simulink model "GFL_Control"  (R2025a)
settings: Solver=FixedStepDiscrete  StartTime=0.0  StopTime=10.0  RelTol=1e-3
undefined symbols (not defined in the file or in its folder): CheckSeconds, Curr_Controllor_Ki, Curr_Controllor_Kp, Curr_Controllor_Max, Curr_Controllor_Min, CurrPIDLimits4d, CurrPIDParams4d, DiscIntNeverNeededParam, MaxGridVolt, MaxGridwFreq, MaxUdcVolt, MinGridwFreq, MinUdcVolt, PLL_f0, PLL_Init_Theta, PLL_Ki, PLL_Kp
libraries: slpidlib x3, spsabctodq0Lib x2, spsdq0toabcLib x1
settings Model: Creator=yucha  LastModifiedBy=yucha
settings OptimizationCC: DefaultParameterBehavior=Inlined  EnhancedBackFolding=on  PassReuseOutputArgsAs=Individual arguments  ZeroExternalMemoryAtStartup=off  ZeroInternalMemoryAtStartup=off  OptimizeBlockOrder=speed  DifferentSizesBufferReuse=on  OptimizationCustomize=off  EfficientTunableParamExpr=on
settings DebuggingCC: ParameterTunabilityLossMsg=error
settings HardwareCC: TargetBitPerPointer=64.0  TargetBitPerSizeT=64.0  TargetBitPerPtrDiffT=64.0  TargetLongLongMode=on  TargetIntDivRoundTo=Zero  TargetEndianess=LittleEndian  TargetWordSize=64.0  TargetHWDeviceType=MATLAB Host  ProdEqTarget=off
settings SFSimCC: MATLABDynamicMemAlloc=off
settings RTWCC: SystemTargetFile=ert_shrlib.tlc  TemplateMakefile=ert_default_tmf  Description=Embedded Coder (host-based shared library target)
settings CodeAppCC: ForceParamTrailComments=on  IgnoreCustomStorageClasses=off  OperatorAnnotations=on  SimulinkDataObjDesc=on  SFDataObjDesc=on  InsertBlockDesc=on
settings STFCustomTargetCC: SystemTargetFile=ert_shrlib.tlc  TargetLangStandard=C99 (ISO)  MultiwordLength=256.0  DynamicStringBufferSize=256.0  GenerateSampleERTMain=on  ParMdlRefBuildCompliant=on  CompOptLevelCompliant=on  CombineOutputUpdateFcns=on  ERTCustomFileBanners=on  SupportContinuousTime=off  SupportNonInlinedSFcns=off  RemoveResetFunc=on  MATLABClassNameForMDSCustomization=Simulink.SoftwareTarget.ERTCustomization  ModelStepFunctionPrototypeControlCompliant=on  GRTInterface=off  UseToolchainInfoCompliant=on
settings ERTTargetCC: ExtModeTransport=0.0  ExtModeStaticAlloc=off  ExtModeMexFile=ext_comm  ExtModeIntrfLevel=Level1  ERTCustomFileTemplate=example_file_process.tlc  TargetLangStandard=C99 (ISO)  GenerateSampleERTMain=on  ConcurrentExecutionCompliant=off  CPPClassGenCompliant=off

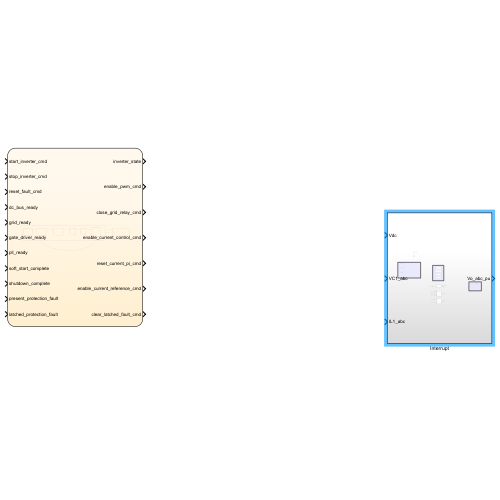
[thumbnail: Simulink's stored preview of the top-level diagram]
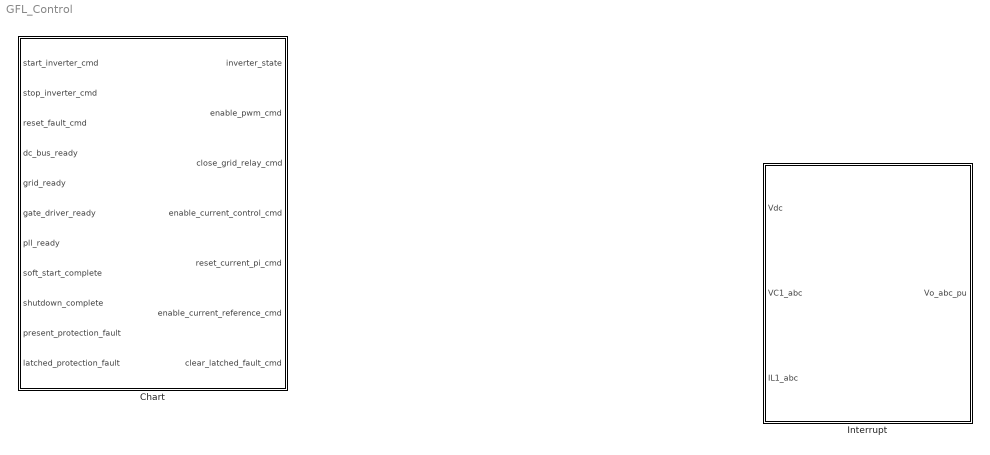
== system GFL_Control ==
  Chart : Stateflow chart  TreatAsAtomicUnit=on
  Interrupt : Subsystem

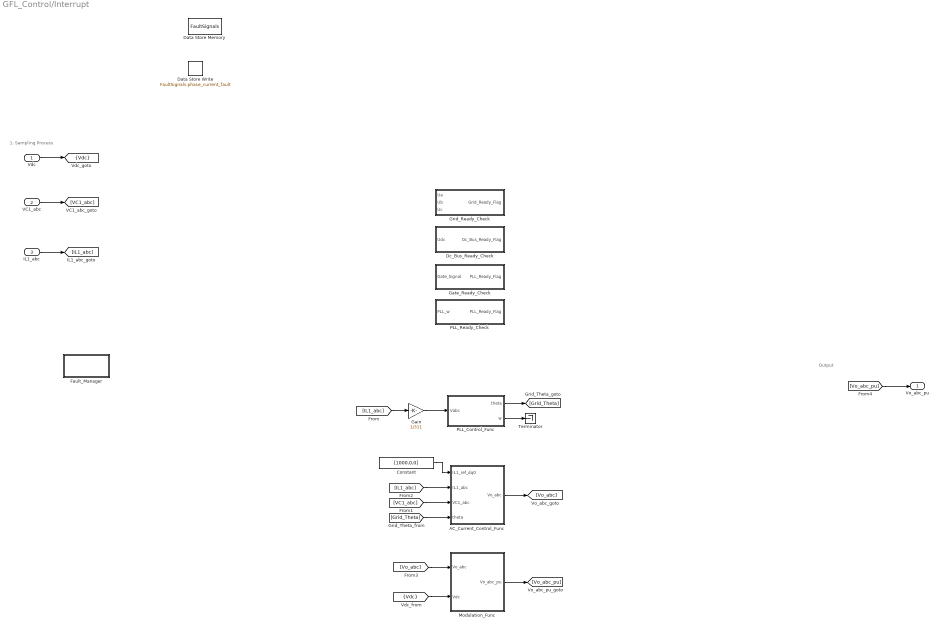
== system GFL_Control/Interrupt ==
  note: 1. Sampling Process
  note: Output
  Vdc : Inport
  VC1_abc : Inport  Port=2
  IL1_abc : Inport  Port=3
  AC_Current_Control_Func : Subsystem  InitFcn=|
      | Curr_Controller_Kp = 1;
      | Curr_Controller_Ki = 1000;
      | Curr_Controller_max = 200;
      | Curr_Controller_min = -200;
  Constant : Constant  Value=[1000,0,0]
  Data Store Memory : DataStoreMemory  DataStoreName=FaultSignals  WriteAfterWriteMsg=warning  ShowAdditionalParam=off  OutDataTypeStr=Bus: FaultSignalsStruct
  Data Store Write : DataStoreWrite  DataStoreName=FaultSignals  DataStoreElements=FaultSignals.phase_current_fault  IndexOptions=Index vector (dialog)  Indices=1  OutputSizes=1
  Dc_Bus_Ready_Check : Subsystem  InitFcn=|
      | MaxUdcVolt = 1200;
      | MinUdcVolt = 650;
      | CheckSeconds = 1;
  Fault_Manager : Subsystem
  Gain : Gain  Gain=1/311
  Gate_Ready_Check : Subsystem  InitFcn=CheckSeconds = 1;
  Grid_Ready_Check : Subsystem
  Modulation_Func : Subsystem  InitFcn=|
      | Curr_Controller_Kp = 1;
      | Curr_Controller_Ki = 1000;
      | Curr_Controller_max = 200;
      | Curr_Controller_min = -200;
  PLL_Control_Func : Subsystem  InitFcn=|
      | PLL_Controller_Kp = 166.0;
      | PLL_Controller_Ki = 25550.0;
      | PLL_Init_Theta = 0;
      | PLL_f0 = 50.0;
  PLL_Ready_Check : Subsystem  InitFcn=|
      | MaxGridwFreq = 100*pi*1.1;
      | MinGridwFreq = 100*pi*0.9;
      | CheckSeconds = 1;
  Terminator : Terminator
  Vo_abc_pu : Outport
  tag scope: Vdc=scoped
  wires:
  VC1_abc/1 -> [VC1_abc]
  IL1_abc/1 -> [IL1_abc]
  Vdc/1 -> [Vdc]
  PLL_Control_Func/2(w) -> Terminator/1
  [Vdc] -> Modulation_Func/2(Vdc)
  Gain/1 -> PLL_Control_Func/1(Vabc)
  [IL1_abc] -> AC_Current_Control_Func/2(IL1_abc)
  [Grid_Theta] -> AC_Current_Control_Func/4(theta)
  [IL1_abc] -> Gain/1
  PLL_Control_Func/1(theta) -> [Grid_Theta]
  [Vo_abc] -> Modulation_Func/1(Vo_abc)
  AC_Current_Control_Func/1(Vo_abc) -> [Vo_abc]
  Modulation_Func/1(Vo_abc_pu) -> [Vo_abc_pu]
  [VC1_abc] -> AC_Current_Control_Func/3(VC1_abc)
  Constant/1 -> AC_Current_Control_Func/1(IL1_ref_dq0)
  [Vo_abc_pu] -> Vo_abc_pu/1

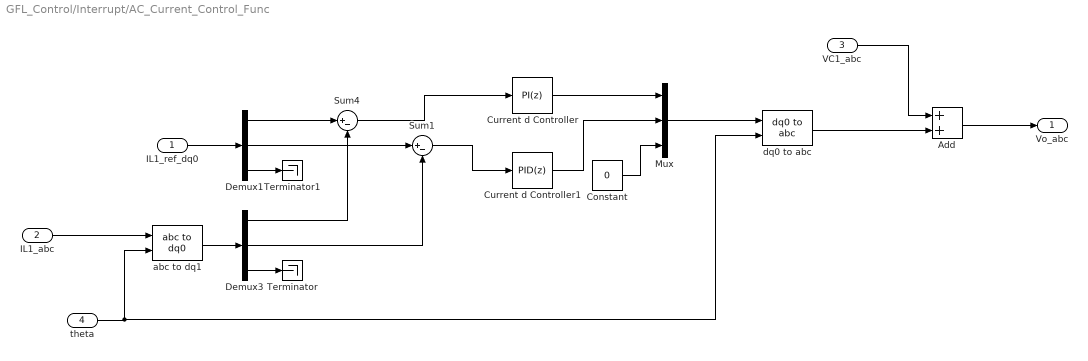
== system GFL_Control/Interrupt/AC_Current_Control_Func ==
  IL1_ref_dq0 : Inport
  IL1_abc : Inport  Port=2
  VC1_abc : Inport  Port=3
  theta : Inport  Port=4
  Add : Sum
  Constant : Constant  Value=0
  Current d Controller : slpidlib/PID Controller  Controller=PI  Form=Parallel  TimeDomain=Discrete-time  UseExternalTs=off  SampleTime=-1  IntegratorMethod=Forward Euler  FilterMethod=Forward Euler  ControllerParametersSource=internal  P=Curr_Controllor_Kp  I=Curr_Controllor_Ki  UseKiTs=on  D=CurrPIDParams4d(3)  UseExternalDerivativeSource=off  N=100  UseFilter=on  TunerSelectOption=Transfer Function Based (PID Tuner App)  InitialConditionSource=internal  InitialConditionForIntegrator=0  InitialConditionForFilter=0  DifferentiatorICPrevScaledInput=0  ExternalReset=none  TrackingMode=off  Kt=1  LimitOutput=on  SatLimitsSource=internal  UpperSaturationLimit=Curr_Controllor_Max  LowerSaturationLimit=Curr_Controllor_Min  LinearizeAsGain=off  AntiWindupMode=clamping  Kb=1  LimitIntegrator=off  UpperIntegratorSaturationLimit=inf  LowerIntegratorSaturationLimit=-inf  POutMin=[]  POutMax=[]  IOutMin=[]  IOutMax=[]  DOutMin=[]  DOutMax=[]  NOutMin=[]  NOutMax=[]  SumOutMin=[]  SumOutMax=[]  SaturationOutMin=[]  SaturationOutMax=[]  PParamMin=[]  PParamMax=[]  IParamMin=[]  IParamMax=[]  DParamMin=[]  DParamMax=[]  NParamMin=[]  NParamMax=[]  KbParamMin=[]  KbParamMax=[]  KtParamMin=[]  KtParamMax=[]  KbOutMin=[]  KbOutMax=[]  KtOutMin=[]  KtOutMax=[]  IntegratorOutMin=[]  IntegratorOutMax=[]  FilterOutMin=[]  FilterOutMax=[]  SumI1OutMin=[]  SumI1OutMax=[]  SumI2OutMin=[]  SumI2OutMax=[]  SumI3OutMin=[]  SumI3OutMax=[]  SumI4OutMin=[]  SumI4OutMax=[]  SumDOutMin=[]  SumDOutMax=[]  DifferentiatorOutMin=[]  DifferentiatorOutMax=[]  FilterDiffOutCoefMin=[]  FilterDiffOutCoefMax=[]  ReciprocalOutMin=[]  ReciprocalOutMax=[]  SumDenOutMin=[]  SumDenOutMax=[]  SumNumOutMin=[]  SumNumOutMax=[]  DivideOutMin=[]  DivideOutMax=[]  UdiffTsProdOutMin=[]  UdiffTsProdOutMax=[]  NTsProdOutMin=[]  NTsProdOutMax=[]  UintegralTsProdOutMin=[]  UintegralTsProdOutMax=[]  UngainTsProdOutMin=[]  UngainTsProdOutMax=[]  ClampingZeroOutDataTypeStr=Inherit: Inherit via back propagation  ClampingZeroOutMin=[]  ClampingZeroOutMax=[]  FilterDenConstantOutDataTypeStr=Inherit: Inherit via back propagation  FilterDenConstantOutMin=[]  FilterDenConstantOutMax=[]  PCopyOutDataTypeStr=Inherit: Inherit via back propagation  PCopyOutMin=[]  PCopyOutMax=[]  NCopyOutDataTypeStr=Inherit: Inherit via back propagation  NCopyOutMin=[]  NCopyOutMax=[]  IntegratorContinuousStateAttributes=''  IntegratorStateMustResolveToSignalObject=off  IntegratorRTWStateStorageClass=Auto  FilterContinuousStateAttributes=''  FilterStateMustResolveToSignalObject=off  FilterRTWStateStorageClass=Auto  ParallelPVariant=InternalParameters  IdealPVariant=Disabled  IVariant=InternalParameters  DVariant=Disabled  IntegratorVariant=Discrete  SatVariant=Enabled  AWVariant=DiscClampingParallel  PCopyVariant=Disabled  TRVariant=Disabled  FdbkBlocksVariant=Forward  IdealPFdbkVariant=Disabled  SatFdbkVariant=Disabled  DerivativeFilterVariant=Disabled  NVariant=Disabled  NCopyVariant=Disabled_SignalSpec  FilterICVariant=Disabled  IntegratorICVariant=InternalICs  ExternalResetVariant=Disabled  TRSumVariant=Passthrough  SumFdbkVariant=Disabled  SumVariant=Sum_PI  TsampFilterVariant=InternalTs  TsampNgainVariant=Passthrough  TsampIntegralVariant=Disabled_SignalSpec  ExternalSaturationOutDataTypeStr=Inherit: Same as second input  DerivativeSourceVariant=Disabled  PreIntVariant=InternalPreInt
      settings: LibrarySourceBlock=simulink/Discrete/Discrete PID Controller
  Current d Controller1 : slpidlib/PID Controller  Controller=PID  Form=Parallel  TimeDomain=Discrete-time  UseExternalTs=off  SampleTime=-1  IntegratorMethod=Forward Euler  FilterMethod=Forward Euler  ControllerParametersSource=internal  P=CurrPIDParams4d(1)  I=CurrPIDParams4d(2)  UseKiTs=off  D=CurrPIDParams4d(3)  UseExternalDerivativeSource=off  N=100  UseFilter=on  TunerSelectOption=Transfer Function Based (PID Tuner App)  InitialConditionSource=internal  InitialConditionForIntegrator=0  InitialConditionForFilter=0  DifferentiatorICPrevScaledInput=0  ExternalReset=none  TrackingMode=off  Kt=1  LimitOutput=on  SatLimitsSource=internal  UpperSaturationLimit=CurrPIDLimits4d(2)  LowerSaturationLimit=CurrPIDLimits4d(1)  LinearizeAsGain=off  AntiWindupMode=clamping  Kb=1  LimitIntegrator=off  UpperIntegratorSaturationLimit=inf  LowerIntegratorSaturationLimit=-inf  POutMin=[]  POutMax=[]  IOutMin=[]  IOutMax=[]  DOutMin=[]  DOutMax=[]  NOutMin=[]  NOutMax=[]  SumOutMin=[]  SumOutMax=[]  SaturationOutMin=[]  SaturationOutMax=[]  PParamMin=[]  PParamMax=[]  IParamMin=[]  IParamMax=[]  DParamMin=[]  DParamMax=[]  NParamMin=[]  NParamMax=[]  KbParamMin=[]  KbParamMax=[]  KtParamMin=[]  KtParamMax=[]  KbOutMin=[]  KbOutMax=[]  KtOutMin=[]  KtOutMax=[]  IntegratorOutMin=[]  IntegratorOutMax=[]  FilterOutMin=[]  FilterOutMax=[]  SumI1OutMin=[]  SumI1OutMax=[]  SumI2OutMin=[]  SumI2OutMax=[]  SumI3OutMin=[]  SumI3OutMax=[]  SumI4OutMin=[]  SumI4OutMax=[]  SumDOutMin=[]  SumDOutMax=[]  DifferentiatorOutMin=[]  DifferentiatorOutMax=[]  FilterDiffOutCoefMin=[]  FilterDiffOutCoefMax=[]  ReciprocalOutMin=[]  ReciprocalOutMax=[]  SumDenOutMin=[]  SumDenOutMax=[]  SumNumOutMin=[]  SumNumOutMax=[]  DivideOutMin=[]  DivideOutMax=[]  UdiffTsProdOutMin=[]  UdiffTsProdOutMax=[]  NTsProdOutMin=[]  NTsProdOutMax=[]  UintegralTsProdOutMin=[]  UintegralTsProdOutMax=[]  UngainTsProdOutMin=[]  UngainTsProdOutMax=[]  ClampingZeroOutDataTypeStr=Inherit: Inherit via back propagation  ClampingZeroOutMin=[]  ClampingZeroOutMax=[]  FilterDenConstantOutDataTypeStr=Inherit: Inherit via back propagation  FilterDenConstantOutMin=[]  FilterDenConstantOutMax=[]  PCopyOutDataTypeStr=Inherit: Inherit via back propagation  PCopyOutMin=[]  PCopyOutMax=[]  NCopyOutDataTypeStr=Inherit: Inherit via back propagation  NCopyOutMin=[]  NCopyOutMax=[]  IntegratorContinuousStateAttributes=''  IntegratorStateMustResolveToSignalObject=off  IntegratorRTWStateStorageClass=Auto  FilterContinuousStateAttributes=''  FilterStateMustResolveToSignalObject=off  FilterRTWStateStorageClass=Auto  ParallelPVariant=InternalParameters  IdealPVariant=Disabled  IVariant=InternalParameters  DVariant=InternalParameters  IntegratorVariant=Discrete  SatVariant=Enabled  AWVariant=DiscClampingParallel  PCopyVariant=Disabled  TRVariant=Disabled  FdbkBlocksVariant=Forward  IdealPFdbkVariant=Disabled  SatFdbkVariant=Disabled  DerivativeFilterVariant=ForwardEulerFilter  NVariant=InternalParameters  NCopyVariant=Disabled  FilterICVariant=InternalICsFilter  IntegratorICVariant=InternalICs  ExternalResetVariant=Disabled  TRSumVariant=Passthrough  SumFdbkVariant=Disabled  SumVariant=Sum_PID  TsampFilterVariant=InternalTs  TsampNgainVariant=Passthrough  TsampIntegralVariant=Disabled_SignalSpec  ExternalSaturationOutDataTypeStr=Inherit: Same as second input  DerivativeSourceVariant=ErrorSignal  PreIntVariant=InternalPreInt
      settings: LibrarySourceBlock=simulink/Discrete/Discrete PID Controller
  Demux1 : Demux  Outputs=3
  Demux3 : Demux  Outputs=3
  Mux : Mux  Inputs=3
  Sum1 : Sum  Inputs=|+-
  Sum4 : Sum  Inputs=|+-
  Terminator : Terminator
  Terminator1 : Terminator
  abc to dq1 : spsabctodq0Lib/abc to dq0  Alignment=Aligned with phase A axis
  dq0 to abc : spsdq0toabcLib/dq0 to abc  Alignment=Aligned with phase A axis
  Vo_abc : Outport
  wires:
  IL1_abc/1 -> abc to dq1/1
  theta/1 -> dq0 to abc/2, abc to dq1/2
  abc to dq1/1 -> Demux3/1
  IL1_ref_dq0/1 -> Demux1/1
  Demux3/3 -> Terminator/1
  Demux1/3 -> Terminator1/1
  Demux1/1 -> Sum4/1
  Demux1/2 -> Sum1/1
  Demux3/1 -> Sum4/2
  Demux3/2 -> Sum1/2
  Sum4/1 -> Current d Controller/1
  Sum1/1 -> Current d Controller1/1
  Current d Controller/1 -> Mux/1
  Current d Controller1/1 -> Mux/2
  Constant/1 -> Mux/3
  Add/1 -> Vo_abc/1
  VC1_abc/1 -> Add/1
  Mux/1 -> dq0 to abc/1
  dq0 to abc/1 -> Add/2

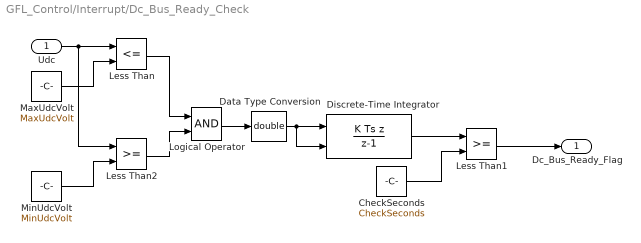
== system GFL_Control/Interrupt/Dc_Bus_Ready_Check ==
  Udc : Inport
  CheckSeconds : Constant  Value=CheckSeconds
  Data Type Conversion : DataTypeConversion  OutDataTypeStr=double  SaturateOnIntegerOverflow=off  RndMeth=Floor
  Discrete-Time Integrator : DiscreteIntegrator  IntegratorMethod=Integration: Backward Euler  ExternalReset=falling  SampleTime=-1  LimitOutput=on  UpperSaturationLimit=100  LowerSaturationLimit=0  ICPrevOutput=DiscIntNeverNeededParam  ICPrevScaledInput=DiscIntNeverNeededParam
  Less Than : RelationalOperator  Operator=<=  OutDataTypeStr=boolean  RndMeth=Simplest  InputSameDT=off
  Less Than1 : RelationalOperator  OutDataTypeStr=boolean  RndMeth=Simplest  InputSameDT=off
  Less Than2 : RelationalOperator  OutDataTypeStr=boolean  RndMeth=Simplest  InputSameDT=off
  Logical Operator : Logic  AllPortsSameDT=off  OutDataTypeStr=boolean
  MaxUdcVolt : Constant  Value=MaxUdcVolt
  MinUdcVolt : Constant  Value=MinUdcVolt
  Dc_Bus_Ready_Flag : Outport
  wires:
  Less Than/1 -> Logical Operator/1
  MaxUdcVolt/1 -> Less Than/2
  CheckSeconds/1 -> Less Than1/2
  Data Type Conversion/1 -> Discrete-Time Integrator/1, Discrete-Time Integrator/2
  Discrete-Time Integrator/1 -> Less Than1/1
  Less Than1/1 -> Dc_Bus_Ready_Flag/1
  Logical Operator/1 -> Data Type Conversion/1
  Udc/1 -> Less Than2/1, Less Than/1
  MinUdcVolt/1 -> Less Than2/2
  Less Than2/1 -> Logical Operator/2

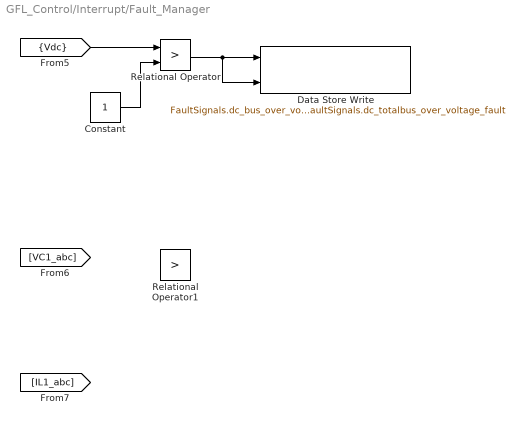
== system GFL_Control/Interrupt/Fault_Manager ==
  Constant : Constant
  Data Store Write : DataStoreWrite  DataStoreName=FaultSignals  DataStoreElements=FaultSignals.dc_bus_over_voltage_fault#FaultSignals.dc_totalbus_over_voltage_fault  IndexOptions=Index vector (dialog)  Indices=1  OutputSizes=1
  Relational Operator : RelationalOperator  Operator=>  OutDataTypeStr=boolean  RndMeth=Simplest  InputSameDT=off
  Relational Operator1 : RelationalOperator  Operator=>  OutDataTypeStr=boolean  RndMeth=Simplest  InputSameDT=off
  wires:
  [Vdc] -> Relational Operator/1
  Constant/1 -> Relational Operator/2
  Relational Operator/1 -> Data Store Write/2, Data Store Write/1

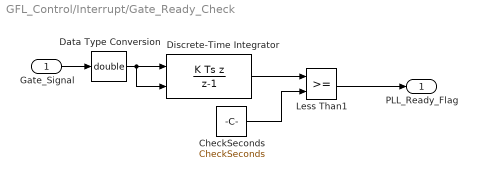
== system GFL_Control/Interrupt/Gate_Ready_Check ==
  Gate_Signal : Inport
  CheckSeconds : Constant  Value=CheckSeconds
  Data Type Conversion : DataTypeConversion  OutDataTypeStr=double  SaturateOnIntegerOverflow=off  RndMeth=Floor
  Discrete-Time Integrator : DiscreteIntegrator  IntegratorMethod=Integration: Backward Euler  ExternalReset=falling  SampleTime=-1  LimitOutput=on  UpperSaturationLimit=100  LowerSaturationLimit=0  ICPrevOutput=DiscIntNeverNeededParam  ICPrevScaledInput=DiscIntNeverNeededParam
  Less Than1 : RelationalOperator  OutDataTypeStr=boolean  RndMeth=Simplest  InputSameDT=off
  PLL_Ready_Flag : Outport
  wires:
  CheckSeconds/1 -> Less Than1/2
  Data Type Conversion/1 -> Discrete-Time Integrator/1, Discrete-Time Integrator/2
  Discrete-Time Integrator/1 -> Less Than1/1
  Less Than1/1 -> PLL_Ready_Flag/1
  Gate_Signal/1 -> Data Type Conversion/1

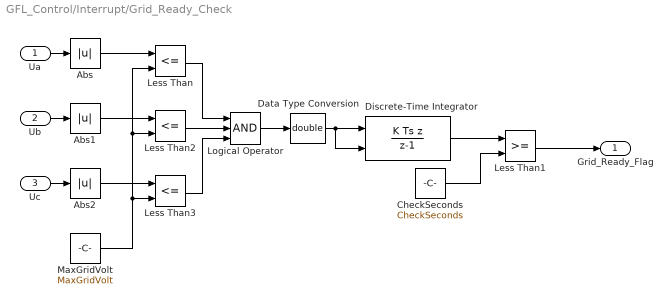
== system GFL_Control/Interrupt/Grid_Ready_Check ==
  Ua : Inport
  Ub : Inport  Port=2
  Uc : Inport  Port=3
  Abs : Abs  SaturateOnIntegerOverflow=off
  Abs1 : Abs  SaturateOnIntegerOverflow=off
  Abs2 : Abs  SaturateOnIntegerOverflow=off
  CheckSeconds : Constant  Value=CheckSeconds
  Data Type Conversion : DataTypeConversion  OutDataTypeStr=double  SaturateOnIntegerOverflow=off  RndMeth=Floor
  Discrete-Time Integrator : DiscreteIntegrator  IntegratorMethod=Integration: Backward Euler  ExternalReset=falling  SampleTime=-1  LimitOutput=on  UpperSaturationLimit=100  LowerSaturationLimit=0  ICPrevOutput=DiscIntNeverNeededParam  ICPrevScaledInput=DiscIntNeverNeededParam
  Less Than : RelationalOperator  Operator=<=  OutDataTypeStr=boolean  RndMeth=Simplest  InputSameDT=off
  Less Than1 : RelationalOperator  OutDataTypeStr=boolean  RndMeth=Simplest  InputSameDT=off
  Less Than2 : RelationalOperator  Operator=<=  OutDataTypeStr=boolean  RndMeth=Simplest  InputSameDT=off
  Less Than3 : RelationalOperator  Operator=<=  OutDataTypeStr=boolean  RndMeth=Simplest  InputSameDT=off
  Logical Operator : Logic  Inputs=3  AllPortsSameDT=off  OutDataTypeStr=boolean
  MaxGridVolt : Constant  Value=MaxGridVolt
  Grid_Ready_Flag : Outport
  wires:
  Abs/1 -> Less Than/1
  Logical Operator/1 -> Data Type Conversion/1
  Less Than1/1 -> Grid_Ready_Flag/1
  Abs1/1 -> Less Than2/1
  Discrete-Time Integrator/1 -> Less Than1/1
  Data Type Conversion/1 -> Discrete-Time Integrator/2, Discrete-Time Integrator/1
  CheckSeconds/1 -> Less Than1/2
  Uc/1 -> Abs2/1
  Ua/1 -> Abs/1
  Abs2/1 -> Less Than3/1
  MaxGridVolt/1 -> Less Than3/2, Less Than2/2, Less Than/2
  Less Than3/1 -> Logical Operator/3
  Less Than2/1 -> Logical Operator/2
  Less Than/1 -> Logical Operator/1
  Ub/1 -> Abs1/1

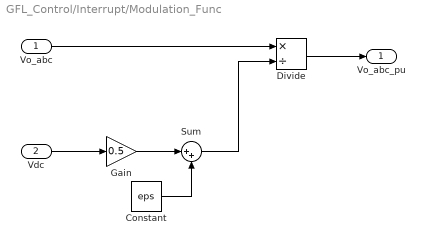
== system GFL_Control/Interrupt/Modulation_Func ==
  Vo_abc : Inport
  Vdc : Inport  Port=2
  Constant : Constant  Value=eps
  Divide : Product  Inputs=*/
  Gain : Gain  Gain=0.5
  Sum : Sum  Inputs=|++
  Vo_abc_pu : Outport
  wires:
  Vo_abc/1 -> Divide/1
  Vdc/1 -> Gain/1
  Gain/1 -> Sum/1
  Constant/1 -> Sum/2
  Sum/1 -> Divide/2
  Divide/1 -> Vo_abc_pu/1

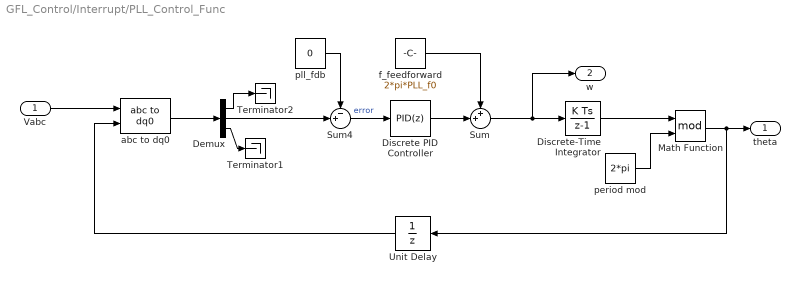
== system GFL_Control/Interrupt/PLL_Control_Func ==
  Vabc : Inport
  Demux : Demux  Outputs=3
  Discrete PID Controller : slpidlib/PID Controller  Controller=PID  Form=Parallel  TimeDomain=Discrete-time  UseExternalTs=off  SampleTime=-1  IntegratorMethod=Forward Euler  FilterMethod=Forward Euler  ControllerParametersSource=internal  P=PLL_Kp  I=PLL_Ki  UseKiTs=off  D=0  UseExternalDerivativeSource=off  N=100  UseFilter=off  TunerSelectOption=Transfer Function Based (PID Tuner App)  InitialConditionSource=internal  InitialConditionForIntegrator=0  InitialConditionForFilter=0  DifferentiatorICPrevScaledInput=0  ExternalReset=none  TrackingMode=off  Kt=1  LimitOutput=on  SatLimitsSource=internal  UpperSaturationLimit=0.2*100*pi  LowerSaturationLimit=-0.2*100*pi  LinearizeAsGain=off  AntiWindupMode=clamping  Kb=1  LimitIntegrator=off  UpperIntegratorSaturationLimit=inf  LowerIntegratorSaturationLimit=-inf  POutMin=[]  POutMax=[]  IOutMin=[]  IOutMax=[]  DOutMin=[]  DOutMax=[]  NOutMin=[]  NOutMax=[]  SumOutMin=[]  SumOutMax=[]  SaturationOutMin=[]  SaturationOutMax=[]  PParamMin=[]  PParamMax=[]  IParamMin=[]  IParamMax=[]  DParamMin=[]  DParamMax=[]  NParamMin=[]  NParamMax=[]  KbParamMin=[]  KbParamMax=[]  KtParamMin=[]  KtParamMax=[]  KbOutMin=[]  KbOutMax=[]  KtOutMin=[]  KtOutMax=[]  IntegratorOutMin=[]  IntegratorOutMax=[]  FilterOutMin=[]  FilterOutMax=[]  SumI1OutMin=[]  SumI1OutMax=[]  SumI2OutMin=[]  SumI2OutMax=[]  SumI3OutMin=[]  SumI3OutMax=[]  SumI4OutMin=[]  SumI4OutMax=[]  SumDOutMin=[]  SumDOutMax=[]  DifferentiatorOutMin=[]  DifferentiatorOutMax=[]  FilterDiffOutCoefMin=[]  FilterDiffOutCoefMax=[]  ReciprocalOutMin=[]  ReciprocalOutMax=[]  SumDenOutMin=[]  SumDenOutMax=[]  SumNumOutMin=[]  SumNumOutMax=[]  DivideOutMin=[]  DivideOutMax=[]  UdiffTsProdOutMin=[]  UdiffTsProdOutMax=[]  NTsProdOutMin=[]  NTsProdOutMax=[]  UintegralTsProdOutMin=[]  UintegralTsProdOutMax=[]  UngainTsProdOutMin=[]  UngainTsProdOutMax=[]  ClampingZeroOutDataTypeStr=Inherit: Inherit via back propagation  ClampingZeroOutMin=[]  ClampingZeroOutMax=[]  FilterDenConstantOutDataTypeStr=Inherit: Inherit via back propagation  FilterDenConstantOutMin=[]  FilterDenConstantOutMax=[]  PCopyOutDataTypeStr=Inherit: Inherit via back propagation  PCopyOutMin=[]  PCopyOutMax=[]  NCopyOutDataTypeStr=Inherit: Inherit via back propagation  NCopyOutMin=[]  NCopyOutMax=[]  IntegratorContinuousStateAttributes=''  IntegratorStateMustResolveToSignalObject=off  IntegratorRTWStateStorageClass=Auto  FilterContinuousStateAttributes=''  FilterStateMustResolveToSignalObject=off  FilterRTWStateStorageClass=Auto  ParallelPVariant=InternalParameters  IdealPVariant=Disabled  IVariant=InternalParameters  DVariant=InternalParameters  IntegratorVariant=Discrete  SatVariant=Enabled  AWVariant=DiscClampingParallel  PCopyVariant=Disabled  TRVariant=Disabled  FdbkBlocksVariant=Forward  IdealPFdbkVariant=Disabled  SatFdbkVariant=Disabled  DerivativeFilterVariant=Differentiator  NVariant=Passthrough  NCopyVariant=Disabled_SignalSpec  FilterICVariant=InternalICsDifferentiator  IntegratorICVariant=InternalICs  ExternalResetVariant=Disabled  TRSumVariant=Passthrough  SumFdbkVariant=Disabled  SumVariant=Sum_PID  TsampFilterVariant=InternalTs  TsampNgainVariant=Passthrough  TsampIntegralVariant=Disabled_SignalSpec  ExternalSaturationOutDataTypeStr=Inherit: Same as second input  DerivativeSourceVariant=ErrorSignal  PreIntVariant=InternalPreInt
      settings: LibrarySourceBlock=simulink/Discrete/Discrete PID Controller
  Discrete-Time Integrator : DiscreteIntegrator  InitialCondition=PLL_Init_Theta  SampleTime=-1  ICPrevOutput=DiscIntNeverNeededParam  ICPrevScaledInput=DiscIntNeverNeededParam
  Math Function : Math  Operator=mod  SignedPower=on
  Sum : Sum  Inputs=++|
  Sum4 : Sum  Inputs=-+|
  Terminator1 : Terminator
  Terminator2 : Terminator
  Unit Delay : UnitDelay  SampleTime=-1  HasFrameUpgradeWarning=on
  abc to dq0 : spsabctodq0Lib/abc to dq0  Alignment=Aligned with phase A axis
  f_feedforward : Constant  Value=2*pi*PLL_f0  SampleTime=0
  period mod : Constant  Value=2*pi  SampleTime=0
  pll_fdb : Constant  Value=0  SampleTime=0
  theta : Outport
  w : Outport  Port=2
  wires:
  f_feedforward/1 -> Sum/1
  Demux/2 -> Sum4/2
  period mod/1 -> Math Function/2
  Unit Delay/1 -> abc to dq0/2
  Discrete PID Controller/1 -> Sum/2
  Demux/3 -> Terminator1/1
  Math Function/1 -> theta/1, Unit Delay/1
  Discrete-Time Integrator/1 -> Math Function/1
  abc to dq0/1 -> Demux/1
  pll_fdb/1 -> Sum4/1
  Sum/1 -> w/1, Discrete-Time Integrator/1
  Vabc/1 -> abc to dq0/1
  Sum4/1 -> Discrete PID Controller/1  "error"
  Demux/1 -> Terminator2/1

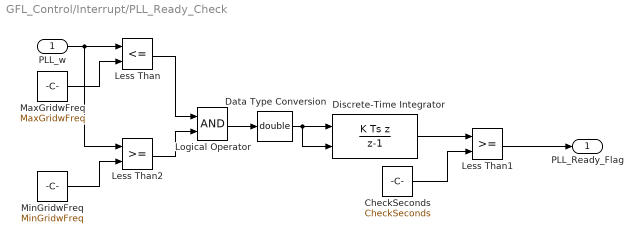
== system GFL_Control/Interrupt/PLL_Ready_Check ==
  PLL_w : Inport
  CheckSeconds : Constant  Value=CheckSeconds
  Data Type Conversion : DataTypeConversion  OutDataTypeStr=double  SaturateOnIntegerOverflow=off  RndMeth=Floor
  Discrete-Time Integrator : DiscreteIntegrator  IntegratorMethod=Integration: Backward Euler  ExternalReset=falling  SampleTime=-1  LimitOutput=on  UpperSaturationLimit=100  LowerSaturationLimit=0  ICPrevOutput=DiscIntNeverNeededParam  ICPrevScaledInput=DiscIntNeverNeededParam
  Less Than : RelationalOperator  Operator=<=  OutDataTypeStr=boolean  RndMeth=Simplest  InputSameDT=off
  Less Than1 : RelationalOperator  OutDataTypeStr=boolean  RndMeth=Simplest  InputSameDT=off
  Less Than2 : RelationalOperator  OutDataTypeStr=boolean  RndMeth=Simplest  InputSameDT=off
  Logical Operator : Logic  AllPortsSameDT=off  OutDataTypeStr=boolean
  MaxGridwFreq : Constant  Value=MaxGridwFreq
  MinGridwFreq : Constant  Value=MinGridwFreq
  PLL_Ready_Flag : Outport
  wires:
  Less Than2/1 -> Logical Operator/2
  MinGridwFreq/1 -> Less Than2/2
  PLL_w/1 -> Less Than/1, Less Than2/1
  Logical Operator/1 -> Data Type Conversion/1
  Less Than1/1 -> PLL_Ready_Flag/1
  Discrete-Time Integrator/1 -> Less Than1/1
  Data Type Conversion/1 -> Discrete-Time Integrator/2, Discrete-Time Integrator/1
  CheckSeconds/1 -> Less Than1/2
  MaxGridwFreq/1 -> Less Than/2
  Less Than/1 -> Logical Operator/1

== stateflow chart GFL_Control/Chart ==
  settings: updateMethod=DISCRETE  sampleTime=1e-3
  state NormalMode
    state Shutdown
      entry:
      inverter_state = 5;
      enable_pwm_cmd = true;
      close_grid_relay_cmd = true;
      enable_current_control_cmd = true;
      reset_current_pi_cmd = false;
      enable_current_reference_cmd = false;
      clear_latched_fault_cmd = false;
    state SoftStart
      entry:
      inverter_state = 3;
      enable_pwm_cmd = true;
      close_grid_relay_cmd = true;
      enable_current_control_cmd = true;
      reset_current_pi_cmd = false;
      enable_current_reference_cmd = true;
      clear_latched_fault_cmd = false;
    state Operation
      entry:
      inverter_state = 4;
      enable_pwm_cmd = true;
      close_grid_relay_cmd = true;
      enable_current_control_cmd = true;
      reset_current_pi_cmd = false;
      enable_current_reference_cmd = true;
      clear_latched_fault_cmd = false;
    state Initialization
      entry:
      inverter_state = 0;
      enable_pwm_cmd = false;
      close_grid_relay_cmd = false;
      enable_current_control_cmd = false;
      reset_current_pi_cmd = true;
      enable_current_reference_cmd = false;
      clear_latched_fault_cmd = false;
    state Standby
      entry:
      inverter_state = 1;
      enable_pwm_cmd = false;
      close_grid_relay_cmd = false;
      enable_current_control_cmd = false;
      reset_current_pi_cmd = true;
      enable_current_reference_cmd = false;
      clear_latched_fault_cmd = false;
    state Synchronization
      entry:
      inverter_state = 2;
      enable_pwm_cmd = false;
      close_grid_relay_cmd = false;
      enable_current_control_cmd = false;
      reset_current_pi_cmd = true;
      enable_current_reference_cmd = false;
      clear_latched_fault_cmd = false;
    (default) -> Initialization
    Synchronization -> SoftStart : [pll_ready ...
        |  && dc_bus_ready ...
        |  && grid_ready ...
        |  && gate_driver_ready]
    Operation -> Shutdown : [stop_inverter_cmd]
    SoftStart -> Operation : [soft_start_complete]
    Initialization -> Standby : [after(100,tick)]
    Standby -> Synchronization : [start_inverter_cmd ...
        |  && dc_bus_ready ...
        |  && grid_ready ...
        |  && gate_driver_ready ...
        |  && ~latched_protection_fault]
  state Fault
    entry:
    inverter_state = -1;
    enable_pwm_cmd = false;
    close_grid_relay_cmd = false;
    enable_current_control_cmd = false;
    reset_current_pi_cmd = true;
    enable_current_reference_cmd = false;
    clear_latched_fault_cmd = false;
    during:
    clear_latched_fault_cmd = reset_fault_cmd && ~present_protection_fault;
  (default) -> NormalMode
  NormalMode -> Fault : [latched_protection_fault]
  Fault -> NormalMode : [~latched_protection_fault && ~present_protection_fault]
  Shutdown -> Standby : [shutdown_complete || after(1000,tick)]
  data: start_inverter_cmd input; stop_inverter_cmd input; reset_fault_cmd input; dc_bus_ready input; grid_ready input; gate_driver_ready input; pll_ready input; soft_start_complete input; shutdown_complete input; present_protection_fault input; latched_protection_fault input; inverter_state output; enable_pwm_cmd output; close_grid_relay_cmd output; enable_current_control_cmd output; reset_current_pi_cmd output; enable_current_reference_cmd output; clear_latched_fault_cmd output
